simulink model "Aeromobile2F"  (R2022b)
settings: Solver=ode1be  StartTime=0.0  StopTime=100  RelTol=1e+10
undefined symbols (not defined in the file or in its folder): Controller1, Controller2
settings Model: Creator=Davide  LastModifiedBy=Davide
settings SolverCC: ConsecutiveZCsStepRelTol=100*128*eps  ZeroCrossControl=EnableAll  ZeroCrossAlgorithm=Adaptive  EnableFixedStepZeroCrossing=on  MaxZcPerStep=200  MaxZcBracketingIterations=100
settings DebuggingCC: IgnoredZcDiagnostic=none  ParameterPrecisionLossMsg=none

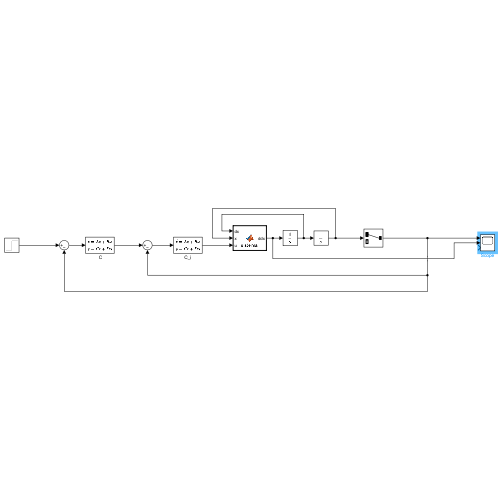
[thumbnail: Simulink's stored preview of the top-level diagram]
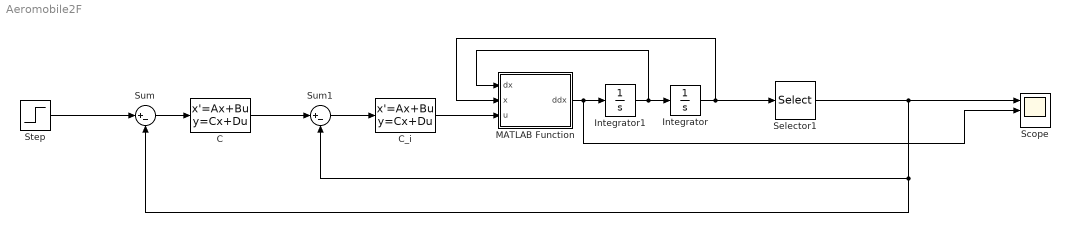
== system Aeromobile2F ==
  " C" : StateSpace  A=Controller2.A  B=Controller2.B  C=Controller2.C  D=Controller2.D  InitialCondition=0
  C_i : StateSpace  A=Controller1.A  B=Controller1.B  C=Controller1.C  D=Controller1.D  InitialCondition=0
  Integrator : Integrator
  Integrator1 : Integrator  InitialCondition=1  IgnoreLimit=on
  MATLAB Function : MATLAB Function  TreatAsAtomicUnit=on
  Scope : Scope  NumInputPorts=3
  Selector1 : Selector  InputPortWidth=2  IndexOptions=Index vector (dialog)  Indices=[1]  OutputSizes=1
  Step : Step  OutDataTypeStr=single  SampleTime=1  VectorParams1D=off  ZeroCross=off
  Sum : Sum  Inputs=|+-
  Sum1 : Sum  Inputs=|+-
  wires:
  Step/1 -> Sum/1
  Integrator/1 -> Selector1/1, MATLAB Function/2(x)
  Integrator1/1 -> Integrator/1, MATLAB Function/1(dx)
  MATLAB Function/1(ddx) -> Scope/2, Integrator1/1
  Sum/1 -> " C"/1
  " C"/1 -> Sum1/1
  Selector1/1 -> Sum/2, Sum1/2, Scope/1
  Sum1/1 -> C_i/1
  C_i/1 -> MATLAB Function/3(u)

== matlab function Aeromobile2F/MATLAB Function ==
  data: dx input; x input; u input; ddx output
function ddx = sistema( dx, x, u)
    % Parametri
    g = 9.81;
    M = 63200;
    J = 235000;
    d = 6.5;
    beta_theta1 = 300;
    beta_theta2 = 450;
    beta_v = 500;
    S = 125;
    rho = 1.5; 

    
    T = u;

    % Stati
    h = x(1);
    theta = x(2);
    dh = dx(1);
    dtheta = dx(2);

    
    D_dh = 0.5 * rho * dh^2 * S;
    gamma_dh = beta_v * dh;

    % Equazioni 
    
    
    ddh = (T * cos(theta) - M * g - D_dh - gamma_dh * sin(theta)^2) / M;
    ddtheta = (T * d * sin(theta) - beta_theta1 * dtheta- beta_theta2 * sin(theta)) / J; 
    
    ddx = [ddh; ddtheta];
end
